simulink model "DC_Motor_Regulator"  (R2023b)
settings: Solver=VariableStepAuto  StartTime=0.0  StopTime=10.0  RelTol=1e-3
StopFcn:
  | show_results_after_sim
values from neighbouring files (symbols this model uses):
  Bm = 0.006126    [parameters.m]
  ke = 1.8    [parameters.m]
  kt = 1.8    [parameters.m]
  Ra = 0.1514    [parameters.m]
  Su = 9.5492    [parameters.m]
libraries: Lab_b x1
settings Model: Creator=Student  LastModifiedBy=Student

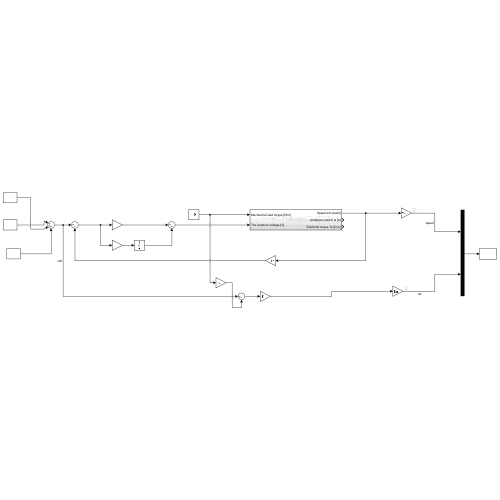
[thumbnail: Simulink's stored preview of the top-level diagram]
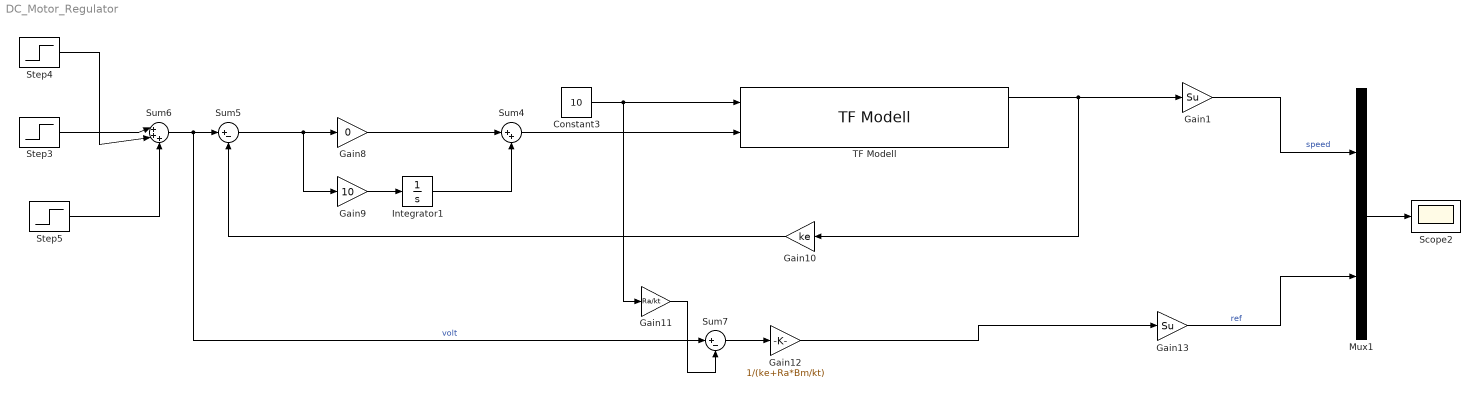
== system DC_Motor_Regulator ==
  Constant3 : Constant  Value=10
  Gain1 : Gain  Gain=Su
  Gain10 : Gain  Gain=ke
  Gain11 : Gain  Gain=Ra/kt
  Gain12 : Gain  Gain=1/(ke+Ra*Bm/kt)
  Gain13 : Gain  Gain=Su
  Gain8 : Gain  Gain=0
  Gain9 : Gain  Gain=10
  Integrator1 : Integrator
  Mux1 : Mux  Inputs=2
  Scope2 : Scope
  Step3 : Step  Time=5.5  After=50  SampleTime=0
  Step4 : Step  Time=8.2  After=150  SampleTime=0
  Step5 : Step  Time=1.1  After=80  SampleTime=0
  Sum4 : Sum  Inputs=|++
  Sum5 : Sum  Inputs=|+-
  Sum6 : Sum  Inputs=|+++
  Sum7 : Sum  Inputs=|+-
  TF Modell : Lab_b/TF Modell  SystemSampleTime=-1  VariantActivationTime=update diagram  AllowFlexibleInterface=on  Latency=0  AutoFrameSizeCalculation=off
      link override Transfer Fcn: Denominator=[La Ra]
  wires:
  Sum4/1 -> TF Modell/2
  Gain10/1 -> Sum5/2
  Mux1/1 -> Scope2/1
  Constant3/1 -> TF Modell/1, Gain11/1
  Gain11/1 -> Sum7/2
  Sum7/1 -> Gain12/1
  Gain12/1 -> Gain13/1
  Gain13/1 -> Mux1/2  "ref"
  Sum6/1 -> Sum5/1, Sum7/1  "volt"
  Step3/1 -> Sum6/1
  Step4/1 -> Sum6/2
  Step5/1 -> Sum6/3
  Integrator1/1 -> Sum4/2
  Gain9/1 -> Integrator1/1
  Gain8/1 -> Sum4/1
  Sum5/1 -> Gain8/1, Gain9/1
  Gain1/1 -> Mux1/1  "speed"
  TF Modell/1 -> Gain1/1, Gain10/1
